simulink model "controller"  (R2022a)
settings: Solver=VariableStepAuto  StartTime=0.0  StopTime=10.0  RelTol=1e-3
settings Model: Creator=eleves  LastModifiedBy=eleves

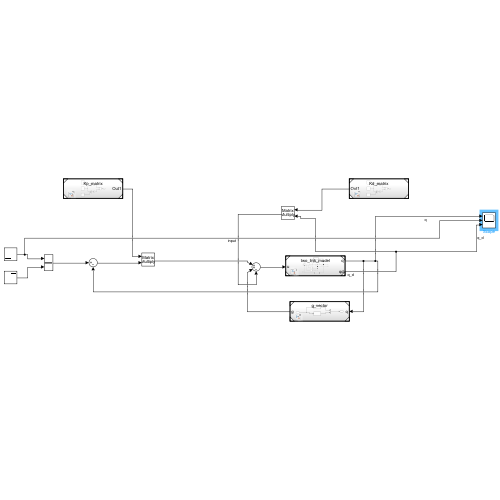
[thumbnail: Simulink's stored preview of the top-level diagram]
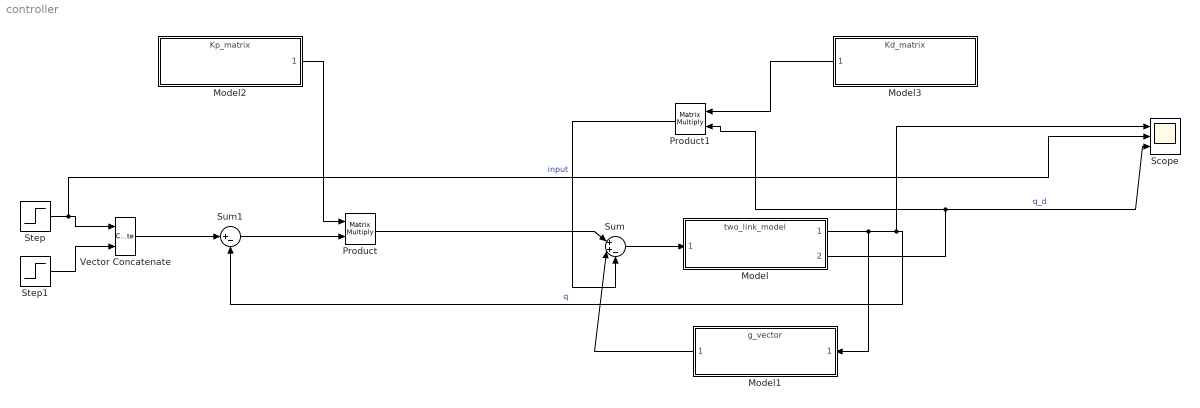
== system controller ==
  Model : ModelReference  ModelNameDialog=two_link_model.slx  SimulationMode=Normal  ModelReferenceVersion=1.3
  Model1 : ModelReference  ModelNameDialog=g_vector.slx  SimulationMode=Normal  ModelReferenceVersion=1.8
  Model2 : ModelReference  ModelNameDialog=Kp_matrix.slx  SimulationMode=Normal  ModelReferenceVersion=1.3
  Model3 : ModelReference  ModelNameDialog=Kd_matrix.slx  SimulationMode=Normal  ModelReferenceVersion=1.2
  Product : Product  Multiplication=Matrix(*)
  Product1 : Product  Multiplication=Matrix(*)
  Scope : Scope  NumInputPorts=3
  Step : Step  After=pi/2  SampleTime=0.1
  Step1 : Step  After=pi/2  SampleTime=0.1
  Sum : Sum  Inputs=|++-
  Sum1 : Sum  Inputs=|+-
  Vector Concatenate : Concatenate
  wires:
  Step/1 -> Scope/2, Vector Concatenate/1  "input"
  Step1/1 -> Vector Concatenate/2
  Sum/1 -> Model/1
  Model1/1 -> Sum/2
  Model/1 -> Sum1/2, Scope/1, Model1/1  "q"
  Model2/1 -> Product/1
  Product/1 -> Sum/1
  Product1/1 -> Sum/3
  Sum1/1 -> Product/2
  Vector Concatenate/1 -> Sum1/1
  Model/2 -> Scope/3, Product1/2  "q_d"
  Model3/1 -> Product1/1
